simulink model "VoiceTransmissionPassband"  (R2018a)
settings: Solver=VariableStepAuto  StartTime=0.0  StopTime=6  RelTol=1e-3
libraries: commanapbnd3 x2, dspvision x2, phasedtxrxlib x2, commchan3 x1, dspsnks4 x1
settings Model: Creator=ASUS  LastModifiedBy=ASUS

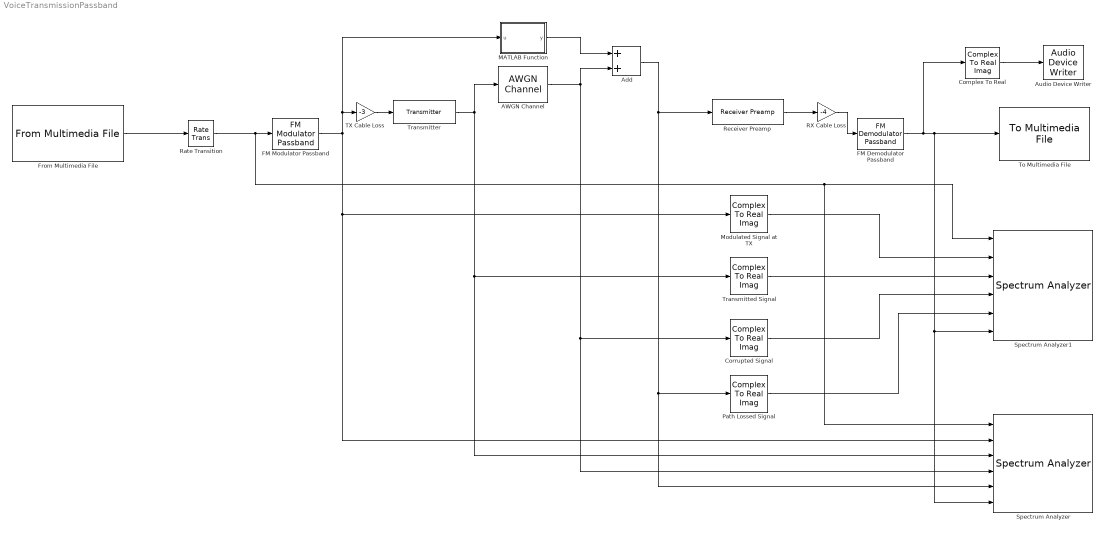
== system VoiceTransmissionPassband ==
  AWGN Channel : commchan3/AWGN Channel  InputProcessing=Columns as channels (frame based)  seed=67  noiseMode="Signal to noise ratio  (Eb/No)"  EbNodB=-20  EsNodB=10  SNRdB=10  bitsPerSym=1  Ps=1  Tsym=1  variance=1
  Add : Sum
  Audio Device Writer : dspsnks4/Audio Device Writer  Driver=DirectSound  Device=Default  InheritSampleRate=on  SampleRate=44100  BitDepth=16-bit integer  BufferSize=4096  NumBuffers=10  DefaultOutputChannelMapping=on  OutputChannelMapping=1:2  OutputNumUnderrunSamples=off  DriverIdx=1  DeviceWarnFlag=''
  Complex To Real : ComplexToRealImag  Output=Real
  Corrupted Signal : ComplexToRealImag  Output=Real
  FM Demodulator Passband : commanapbnd3/FM Demodulator Passband  Fc=50e9  Ph=0  Kc=4000  Ho=100
      settings: SourceProductName=Communications System Toolbox  SourceProductBaseCode=CM
  FM Modulator Passband : commanapbnd3/FM Modulator Passband  Fc=50e9  Ph=0  Kc=4000
      settings: SourceProductName=Communications System Toolbox  SourceProductBaseCode=CM
  From Multimedia File : dspvision/From Multimedia File  inputFilename=C:\Users\ASUS\Desktop\GitRepos\RF-Propagation-Model\RFPL Modelling\code\voice.wav  loop=on  numPlays=inf  outputStreams=Audio only  videoDataType=single  audioDataType=double  inheritSampleTime=on  userDefinedSampleTime=1/7999  noAudioOutput=off  isIntensityVideo=off  fourcc=RGB  colorVideoFormat=Separate color signals  outputEOF=off  dataOrg=Column-major  audioFrameSize=1024  computeAudioFrameSize=off  outSamplingMode=Sample based
      settings: SourceProductBaseCode=VP
  MATLAB Function : MATLAB Function  TreatAsAtomicUnit=on
  Modulated Signal at TX : ComplexToRealImag  Output=Real
  Path Lossed Signal : ComplexToRealImag  Output=Real
  RX Cable Loss : Gain  Gain=-4
  Rate Transition : RateTransition
  Receiver Preamp : phasedtxrxlib/Receiver Preamp  Gain=24.77  LossFactor=0  NoiseMethod=Noise temperature  NoiseFigure=0  ReferenceTemperature=290  SampleRateFromInputCheckbox=on  SampleRate=1e6  NoisePower=0  EnableInputPort=off  PhaseNoiseInputPort=off  SeedSource=Property  Seed=randi(65535,1)  SimulateUsing=Interpreted execution
      settings: SourceProductName=Phased Array System Toolbox  SourceProductBaseCode=AR
  Spectrum Analyzer : SpectrumAnalyzer  NumInputPorts=6  IsFrequencyInputMode=1
  Spectrum Analyzer1 : SpectrumAnalyzer  NumInputPorts=6
  "TX Cable Loss " : Gain  Gain=-3
  To Multimedia File : dspvision/To Multimedia File  outputFilename=C:\Users\ASUS\Desktop\GitRepos\RF-Propagation-Model\RFPL Modelling\code\output.wav  streamSelection=Audio only  videoCompressor=None (uncompressed)  audioCompressor=None (uncompressed)  imagePorts=Separate color signals  fileType=WAV  audioDatatype=16-bit integer  fourcc=RGB  videoQuality=75  mj2000CompFactor=10
      settings: SourceProductName=Computer Vision System Toolbox  SourceProductBaseCode=VP
  "Transmitted Signal " : ComplexToRealImag  Output=Real
  Transmitter : phasedtxrxlib/Transmitter  PeakPower=50000  Gain=30  LossFactor=0  InUseOutputPort=off  CoherentOnTransmit=on  PhaseNoiseOutputPort=off  SeedSource=Property  Seed=randi(65535,1)  SimulateUsing=Interpreted execution
      settings: SourceProductName=Phased Array System Toolbox  SourceProductBaseCode=AR
  wires:
  FM Modulator Passband/1 -> Spectrum Analyzer/2, Modulated Signal at TX/1, MATLAB Function/1(u), "TX Cable Loss "/1
  FM Demodulator Passband/1 -> Complex To Real/1, Spectrum Analyzer/6, Spectrum Analyzer1/6, To Multimedia File/1
  RX Cable Loss/1 -> FM Demodulator Passband/1
  "TX Cable Loss "/1 -> Transmitter/1
  Receiver Preamp/1 -> RX Cable Loss/1
  Corrupted Signal/1 -> Spectrum Analyzer1/4
  AWGN Channel/1 -> Spectrum Analyzer/4, Corrupted Signal/1, Add/2
  Modulated Signal at TX/1 -> Spectrum Analyzer1/2
  "Transmitted Signal "/1 -> Spectrum Analyzer1/3
  Path Lossed Signal/1 -> Spectrum Analyzer1/5
  MATLAB Function/1(y) -> Add/1
  Add/1 -> Spectrum Analyzer/5, Path Lossed Signal/1, Receiver Preamp/1
  Complex To Real/1 -> Audio Device Writer/1
  Transmitter/1 -> "Transmitted Signal "/1, Spectrum Analyzer/3, AWGN Channel/1
  From Multimedia File/1 -> Rate Transition/1
  Rate Transition/1 -> FM Modulator Passband/1, Spectrum Analyzer/1, Spectrum Analyzer1/1

== matlab function VoiceTransmissionPassband/MATLAB Function ==
  data: u input; y output
function y = fcn(u)

%Variable Definition
f_GHz = 50;    %Carrier Frequency
freq = f_GHz*1e9 + abs(fft(u))';
range = 10e3;  % Distance between transmitter and receiver in m
rainrate = 20; % Rain rate in mm/h
elev = 0;      % Elevation angle of the propagation path
tau = 0;       % Polarization tilt angle of the signal
temp = 31;     % Ambient Temperature in celcious
dens = 0.5;    % Liquid Water Density in g/m^3
rou = 30.4;    % Water Vapor Density in g/m^3 
p =  101325;   % Atmospheric Pressure in Pa at sea level

freeSpaceLoss = 112.44778322 + 20*log10(freq*1e-9);
rainAttenuation = rainpl(range,freq,rainrate,elev,tau);
fogAttenuation = fogpl(range,freq,temp,dens);
gasAttenuation = gaspl(range,freq,temp, p, rou);

% Calculating total Attenuation
Totalpathloss = freeSpaceLoss + rainAttenuation + ...
                fogAttenuation +gasAttenuation;
            
y = (-1)*Totalpathloss';
